simulink model "test_interpolation"  (R2023b)
settings: Solver=FixedStepAuto  StartTime=0.0  StopTime=1  FixedStep=1  RelTol=1e-3
libraries: nav_lib x1
settings Model: Creator=brent  LastModifiedBy=brent

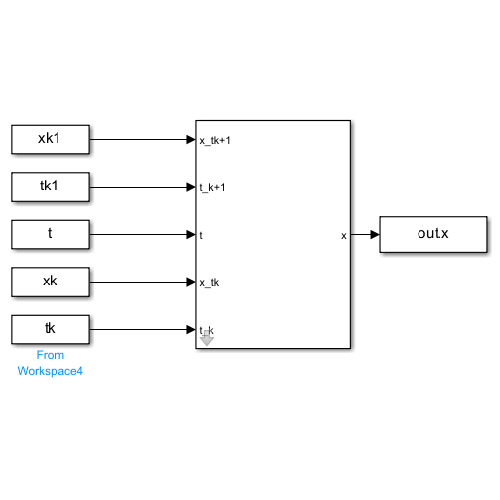
[thumbnail: Simulink's stored preview of the top-level diagram]
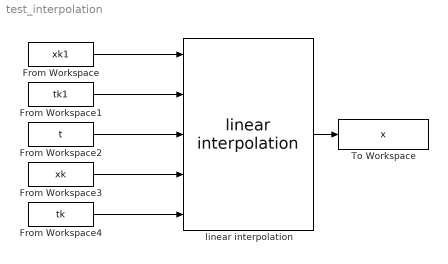
== system test_interpolation ==
  From Workspace : FromWorkspace  VariableName=xk1
  From Workspace1 : FromWorkspace  VariableName=tk1
  From Workspace2 : FromWorkspace  VariableName=t
  From Workspace3 : FromWorkspace  VariableName=xk
  From Workspace4 : FromWorkspace  VariableName=tk
  To Workspace : ToWorkspace  VariableName=x  SampleTime=-1
      settings: Save2DSignal=2-D array (concatenate along first dimension)
  linear interpolation : nav_lib/linear interpolation
      settings: SourceProductName=Navigation library
  wires:
  From Workspace/1 -> linear interpolation/1
  From Workspace1/1 -> linear interpolation/2
  From Workspace2/1 -> linear interpolation/3
  From Workspace3/1 -> linear interpolation/4
  From Workspace4/1 -> linear interpolation/5
  linear interpolation/1 -> To Workspace/1
